simulink model "sintonizacao_pi"  (R2012b)
settings: Solver=ode45  StartTime=0.0  StopTime=3  MaxStep=1e-4  RelTol=1e-3
undefined symbols (not defined in the file): sigbuilder_block
libraries: BLDC x6, simulink x1
settings Model: Creator=h3now  LastModifiedBy=h3now

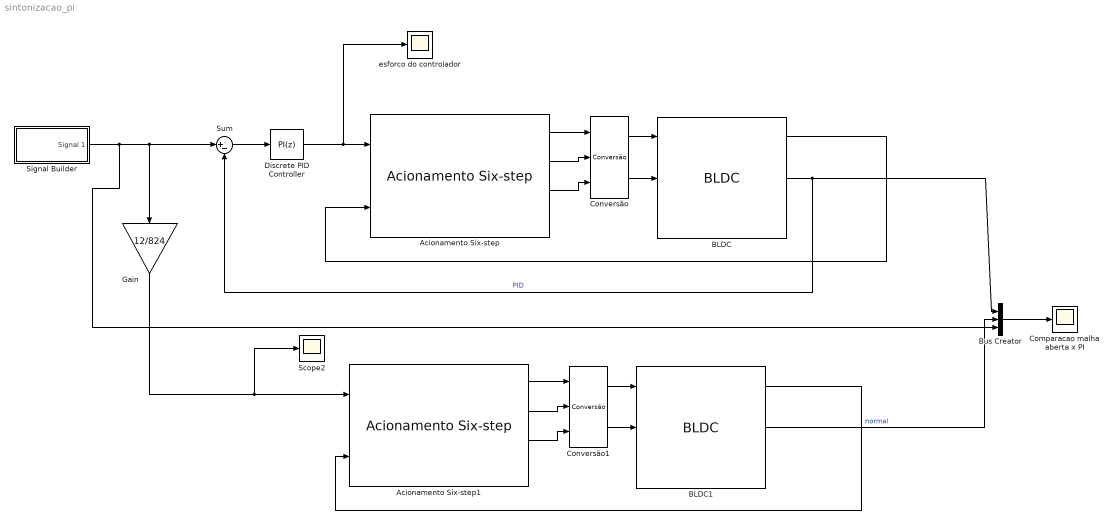
== system sintonizacao_pi ==
  Acionamento Six-step : BLDC/Acionamento Six-step  P=8
  Acionamento Six-step1 : BLDC/Acionamento Six-step  P=8
  BLDC : BLDC/BLDC  J=1.39e-6  R=10.1/2  L=2.04/2000  P=8  Kt=15.7e-3/1.19  Ke=15.7e-3/1.19  Kd=0  F_stick=0.001  F_slip=0.001  default_fcem=on  fcem_a=fcem_a  fcem_b=fcem_b  fcem_c=fcem_c
  BLDC1 : BLDC/BLDC  J=1.39e-6  R=10.1/2  L=2.04/2000  P=8  Kt=15.7e-3/1.19  Ke=15.7e-3/1.19  Kd=0  F_stick=0.001  F_slip=0.001  default_fcem=on  fcem_a=fcem_a  fcem_b=fcem_b  fcem_c=fcem_c
  Bus Creator : BusCreator  Inputs=3
  Comparacao malha aberta x PI : Scope
      settings: ShowLegends=on  YMin=-500  YMax=550
  Conversão : BLDC/Conversão
  Conversão1 : BLDC/Conversão
  Discrete PID Controller : simulink/Continuous/PID Controller  Controller=PI  TimeDomain=Discrete-time  SampleTime=0.01  IntegratorMethod=Forward Euler  FilterMethod=Forward Euler  Form=Parallel  P=0.109710962979121  I=1.86919880777628  D=-0.000461625975032197  N=33.540542961083  InitialConditionSource=internal  InitialConditionForIntegrator=0  InitialConditionForFilter=0  ExternalReset=none  LimitOutput=on  UpperSaturationLimit=12  LowerSaturationLimit=-12  LinearizeAsGain=off  AntiWindupMode=clamping  Kb=1  TrackingMode=off  Kt=1  PParamMin=[]  PParamMax=[]  IParamMin=[]  IParamMax=[]  DParamMin=[]  DParamMax=[]  NParamMin=[]  NParamMax=[]  KbParamMin=[]  KbParamMax=[]  KtParamMin=[]  KtParamMax=[]  POutMin=[]  POutMax=[]  IOutMin=[]  IOutMax=[]  DOutMin=[]  DOutMax=[]  NOutMin=[]  NOutMax=[]  KbOutMin=[]  KbOutMax=[]  KtOutMin=[]  KtOutMax=[]  IntegratorOutMin=[]  IntegratorOutMax=[]  FilterOutMin=[]  FilterOutMax=[]  SumOutMin=[]  SumOutMax=[]  SumI1OutMin=[]  SumI1OutMax=[]  SumI2OutMin=[]  SumI2OutMax=[]  SumI3OutMin=[]  SumI3OutMax=[]  SumDOutMin=[]  SumDOutMax=[]  SaturationOutMin=[]  SaturationOutMax=[]  IntegratorContinuousStateAttributes=''  IntegratorStateMustResolveToSignalObject=off  IntegratorRTWStateStorageClass=Auto  FilterContinuousStateAttributes=''  FilterStateMustResolveToSignalObject=off  FilterRTWStateStorageClass=Auto
  Gain : Gain  Gain=12/824
  Scope2 : Scope
      settings: YMin=7.284  YMax=7.2935  SaveName=ScopeData2
  Signal Builder : Subsystem  Tag=STV Subsys  LoadFcn=sigbuilder_block('load');  StartFcn=sigbuilder_block('start');  StopFcn=sigbuilder_block('stop');  ClipboardFcn=sigbuilder_block('clipboard');  mask(Sigbuilder block){}
      mask help: Simulink:masks:SigbuilderBlock_MD
      mask init:
      | if ~strcmp(get_param(bdroot(gcbh),'SimulationStatus'),'stopped') tuvar = sigbuilder_block('maskInit'); end
      settings: CopyFcn=sigbuilder_block('copy');  DeleteFcn=sigbuilder_block('delete');  ModelCloseFcn=sigbuilder_block('modelClose');  PreSaveFcn=sigbuilder_block('preSave');  PauseFcn=sigbuilder_block('pause');  ContinueFcn=sigbuilder_block('continue');  NameChangeFcn=sigbuilder_block('namechange');  OpenFcn=sigbuilder_block('open',[437.25 199.5 550.5 399.75 ]);  CloseFcn=sigbuilder_block('close');
      mask Display: plot(0, 0, 100, 100,[2, 2, 32, 32, 2], [68, 8, 8, 68, 68],[32, 2], [38, 38], [32, 19, 2],[53, 60, 44], [32, 17, 17, 2],[16, 16, 31, 31]);txt = getActiveGroup(gcbh);text(2, 100, txt,'verticalAlignment', 'top');
  Sum : Sum  Inputs=|+-
  esforco do controlador : Scope
      settings: YMin=7.284  YMax=7.2935
  wires:
  Conversão/1 -> BLDC/1
  Conversão/2 -> BLDC/2
  Acionamento Six-step/1 -> Conversão/1
  Acionamento Six-step/2 -> Conversão/2
  Acionamento Six-step/3 -> Conversão/3
  BLDC/2 -> Sum/2, Bus Creator/1  "PID"
  BLDC/1 -> Acionamento Six-step/2
  Sum/1 -> Discrete PID Controller/1
  Discrete PID Controller/1 -> esforco do controlador/1, Acionamento Six-step/1
  Conversão1/1 -> BLDC1/1
  Conversão1/2 -> BLDC1/2
  Acionamento Six-step1/1 -> Conversão1/1
  Acionamento Six-step1/2 -> Conversão1/2
  Acionamento Six-step1/3 -> Conversão1/3
  BLDC1/2 -> Bus Creator/2  "normal"
  Gain/1 -> Scope2/1, Acionamento Six-step1/1
  BLDC1/1 -> Acionamento Six-step1/2
  Bus Creator/1 -> Comparacao malha aberta x PI/1
  Signal Builder/1(Signal 1) -> Bus Creator/3, Sum/1, Gain/1

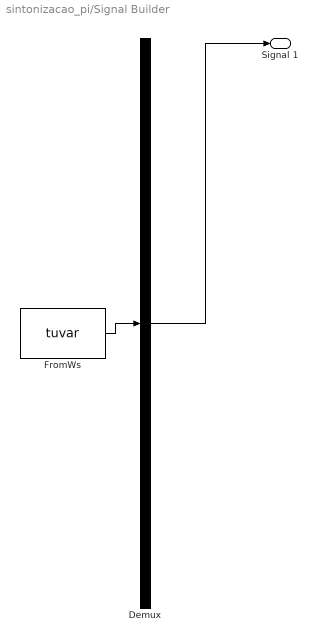
== system sintonizacao_pi/Signal Builder ==
  Demux : Demux  Tag=STV Demux  Outputs=1
  FromWs : FromWorkspace  Tag=STV FromWs  VariableName=tuvar  SampleTime=0
      SigBuilderData=|
      | common.afterFinalStr = 'Extrapolate'
      | common.sampleTime = 0
      | dataSet.timeRange = [0 10]
      | dataSet.name = 'Group 1'
      | sbobj.Groups.Name = 'Group 1'
      | sbobj.Groups.Signals.Name = 'Signal 1'
      | sbobj.Groups.Signals.XData = [0 1 1.01 2 2 3 10]
      | sbobj.Groups.Signals.YData = [500 500 -500 -500 0 0 0]
  Signal 1 : Outport  Tag=STV Outport
  wires:
  Demux/1 -> Signal 1/1
  FromWs/1 -> Demux/1
